simulink model "SerieRuidoEntrada1"  (Simulink 7.2)
settings: Solver=ode3  StartTime=0.0  StopTime=15  FixedStep=10^-3  RelTol=1e-3
values from neighbouring files (symbols this model uses):
  FTf = 1/mag*FTfp    [Filtros.m]    (also in RuidoFiltroN.m)
  FTf2 = 1/mag2*FTfp2    [Filtros.m]    (also in RuidoFiltroN.m)
  FTf3 = 1/mag3*FTfp3    [Filtros.m]
libraries: simulink x1
settings Model: Creator=Ferdinando  LastModifiedBy=FVOliveira
settings DebuggingCC: StrictBusMsg=ErrorLevel1

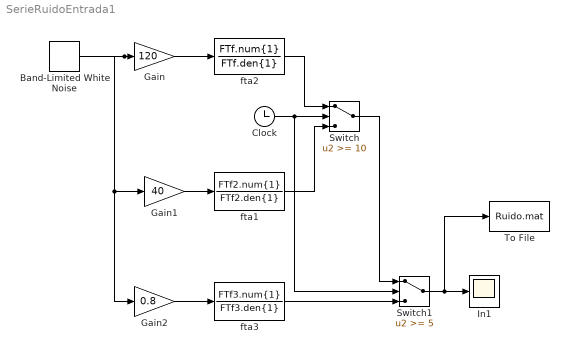
== system SerieRuidoEntrada1 ==
  Band-Limited White Noise : simulink/Sources/Band-Limited White Noise  SystemSampleTime=-1  Cov=[3.163*10^-5]  Ts=10^-3  seed=[23341]
  Clock : Clock
      settings: Decimation=10
  Gain : Gain  Gain=120  ParameterDataType=fixdt(1, 16)  ParameterScaling=2^0  OutDataType=fixdt(1, 16)  OutScaling=2^0
  Gain1 : Gain  Gain=40  ParameterDataType=fixdt(1, 16)  ParameterScaling=2^0  OutDataType=fixdt(1, 16)  OutScaling=2^0
  Gain2 : Gain  Gain=0.8  ParameterDataType=fixdt(1, 16)  ParameterScaling=2^0  OutDataType=fixdt(1, 16)  OutScaling=2^0
  In1 : Scope
      settings: SaveName=Rand3and
  Switch : Switch  Threshold=10  OutDataType=fixdt(1, 16)  OutScaling=2^0
  Switch1 : Switch  Threshold=5  OutDataType=fixdt(1, 16)  OutScaling=2^0
  To File : ToFile  Filename=Ruido.mat  MatrixName=Ruido
  fta1 : TransferFcn  Numerator=FTf2.num{1}  Denominator=FTf2.den{1}
  fta2 : TransferFcn  Numerator=FTf.num{1}  Denominator=FTf.den{1}
  fta3 : TransferFcn  Numerator=FTf3.num{1}  Denominator=FTf3.den{1}
  wires:
  Band-Limited White Noise/1 -> Gain1/1, Gain2/1, Gain/1
  fta2/1 -> Switch/1
  Clock/1 -> Switch/2, Switch1/2
  fta1/1 -> Switch/3
  Switch/1 -> Switch1/1
  fta3/1 -> Switch1/3
  Switch1/1 -> In1/1, To File/1
  Gain/1 -> fta2/1
  Gain1/1 -> fta1/1
  Gain2/1 -> fta3/1
